simulink model "Test_control_Openfast"  (R2021b)
settings: Solver=ode4  StartTime=0.0  StopTime=TMax  FixedStep=DT  MaxStep=DT  RelTol=1e-3  EnableMultiTasking=on
values from neighbouring files (symbols this model uses):
  Bdt = 4.83e8    (= 483000000)    [Run_Test_control_Openfast.m]
  GBRatio = 87,965    [Run_Test_control_Openfast.m]
  Lambda_opt = 6.443736553192139    (= 6.44373655319)    [Run_Test_control_Openfast.m]
undefined symbols (not defined in the file or in its folder): OutList, strmatch
settings Model: Creator=bjonkman  LastModifiedBy=manip
settings SolverCC: AlgebraicLoopSolver=TrustRegion
settings DataIOCC: LimitDataPoints=on  SignalLoggingSaveFormat=ModelDataLogs  SaveOutput=off  SaveTime=off  ReturnWorkspaceOutputs=off  SignalLoggingName=sigsOut
settings OptimizationCC: ExpressionDepthLimit=2147483647  LifeSpan=inf
settings DebuggingCC: SaveWithParameterizedLinksMsg=none  UnderspecifiedInitializationDetection=Classic  MergeDetectMultiDrivingBlocksExec=none  SignalResolutionControl=TryResolveAllWithWarning  MultiTaskDSMMsg=warning  MultiTaskCondExecSysMsg=none  MultiTaskRateTransMsg=warning  FcnCallInpInsideContextMsg=warning  StateNameClashWarn=warning  SFUnexpectedBacktrackingDiag=warning  SFNoUnconditionalDefaultTransitionDiag=warning  SFExecutionAtInitializationDiag=none  SFMachineParentedDataDiag=warning  ArithmeticOperatorsInVariantConditions=warning
settings HardwareCC: ProdBitPerPointer=32  ProdBitPerSizeT=32  ProdBitPerPtrDiffT=32  ProdLargestAtomicFloat=None  ProdIntDivRoundTo=Undefined  ProdEndianess=Unspecified  ProdWordSize=32  ProdHWDeviceType=32-bit Generic  TargetUnknown=on
settings ModelReferenceCC: PropagateSignalLabelsOutOfModel=off
settings SFSimCC: SimUseLocalCustomCode=off  CustomCodeUndefinedFunction=UseInterfaceOnly
settings RTWCC: RTWUseLocalCustomCode=off
settings CodeAppCC: StateflowObjectComments=on
settings GRTTargetCC: TargetLangStandard=C89/C90 (ANSI)  CombineOutputUpdateFcns=off  GRTInterface=on
settings ConfigComp: CovMetricSettings=dw  CovSaveCumulativeToWorkspaceVar=on  CovSaveSingleToWorkspaceVar=on  CovExternalEMLEnable=off

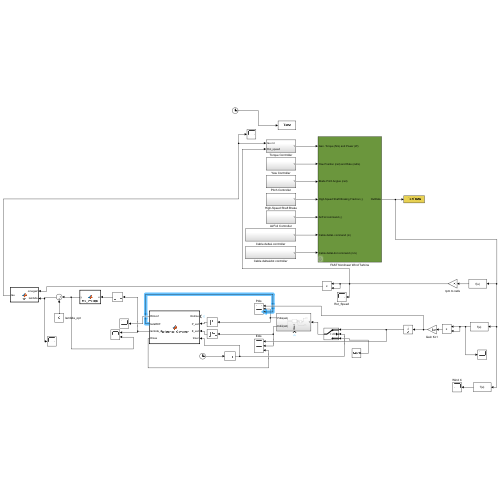
[thumbnail: Simulink's stored preview of the top-level diagram]
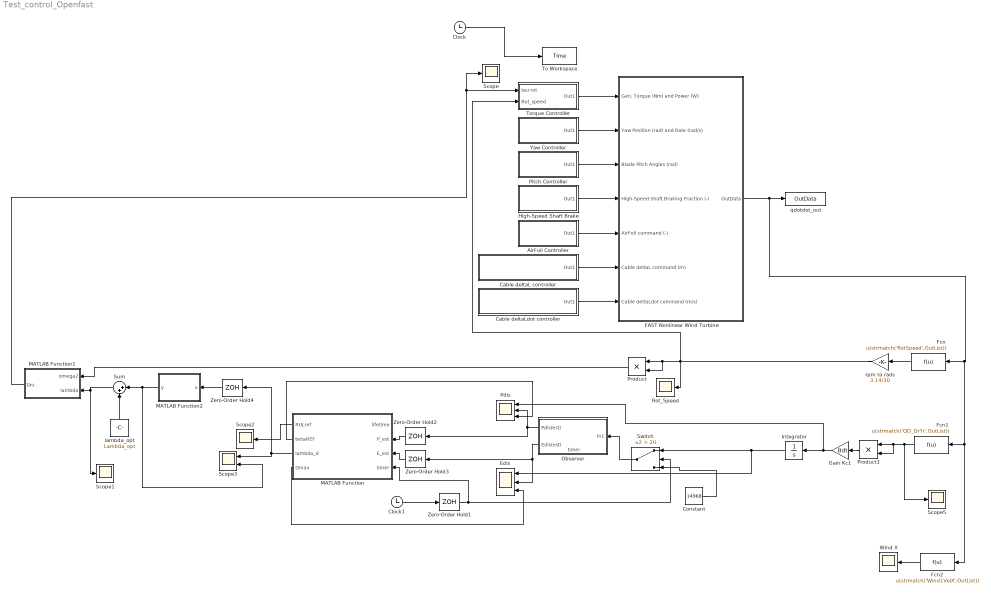
== system Test_control_Openfast ==
  AirFoil Controller : Subsystem
  Cable deltaL controller : Subsystem
  Cable deltaLdot controller : Subsystem
  Clock : Clock
  Clock1 : Clock
  Constant : Constant  Value=14968
  Edis : Scope  NumInputPorts=3
  FAST Nonlinear Wind Turbine : Subsystem  mask(FAST Nonlinear Wind Turbine){}
      mask help: This block contains the FAST S-Function.
      mask init:
      | clear FAST_SFunc
  Fcn : Fcn  Expr=u(strmatch('RotSpeed',OutList))
  Fcn1 : Fcn  Expr=u(strmatch('QD_DrTr',OutList))
  Fcn2 : Fcn  Expr=u(strmatch('Wind1VelX',OutList))
  Gain Kc1 : Gain  Gain=Bdt
  High-Speed Shaft Brake : Subsystem
  Integrator : Integrator
  MATLAB Function : MATLAB Function  TreatAsAtomicUnit=on
  MATLAB Function1 : MATLAB Function  TreatAsAtomicUnit=on
  MATLAB Function2 : MATLAB Function  TreatAsAtomicUnit=on
  Observer : Subsystem
      settings: PortSchema="{\"entries\":[{\"content\":{\"sides\":[{\"content\":{\"connectorIds\":[\"In1\"]},\"type\":\"ConnectorPlacement.EquallySpacedRectSide\",\"uuid\":\"45431176-5fec-4c34-81d0-337d69ca9793\"},{\"content\":{\"connectorIds\":[\"Out1\",\"Out2\"],\"side\":\"RIGHT\"},\"type\":\"ConnectorPlacement.EquallySpacedRectSide\",\"uuid\":\"e3405e5b-b033-438f-b194-16e352d87631\"},{\"content\":{\"connectorIds\":[],\"side\":\"TOP\"},\"type\":\"ConnectorPlacement.EquallySpacedRectSide\",\"uuid\":\"639d392e-3d04-4bae-853f-d03d3019a83c\"},{\"content\":{\"connectorIds\":[\"In2\"],\"side\":\"BOTTOM\"},\"type\":\"ConnectorPlacement.EquallySpacedRectSide\",\"uuid\":\"dfd43518-24a4-48aa-b01e-37d00dba9bed\"}]},\"type\":\"ConnectorPlacement.EquallySpacedConnector\",\"uuid\":\"4ac14b68-7214-4060-a02f-334c8370bb31\"}],\"packageUris\":[\"http://schema.mathworks.com/mf0/Connector/R2020b\"],\"version\":\"1.0\"}"
  Pdis : Scope  NumInputPorts=3
  Pitch Controller : Subsystem
  Product : Product
  Product1 : Product
  Rot_Speed : Scope
  Scope{,1..2,5} (4 alike) : Scope
  Scope3 : Scope  NumInputPorts=2
  Sum : Sum  Inputs=|++
  Switch : Switch  Criteria=u2 > Threshold  Threshold=20
  To Workspace : ToWorkspace  VariableName=Time  SampleTime=-1
  Torque Controller : Subsystem
  Wind X : Scope
  Yaw Controller : Subsystem
  Zero-Order Hold1 : ZeroOrderHold
  Zero-Order Hold2 : ZeroOrderHold
  Zero-Order Hold3 : ZeroOrderHold
  Zero-Order Hold4 : ZeroOrderHold  SampleTime=0.005
  "lambda_opt\t" : Constant  Value=Lambda_opt
  qdotdot_out : ToWorkspace  VariableName=OutData  SampleTime=-1
  rpm to rads : Gain  Gain=3.14/30
  wires:
  Clock/1 -> To Workspace/1
  Torque Controller/1(Out1) -> FAST Nonlinear Wind Turbine/1(Gen. Torque (Nm) and Power (W))
  Yaw Controller/1(Out1) -> FAST Nonlinear Wind Turbine/2(Yaw Position (rad) and Rate (rad/s))
  Pitch Controller/1(Out1) -> FAST Nonlinear Wind Turbine/3(Blade Pitch Angles (rad))
  High-Speed Shaft Brake/1(Out1) -> FAST Nonlinear Wind Turbine/4(High-Speed Shaft Braking Fraction (-))
  AirFoil Controller/1(Out1) -> FAST Nonlinear Wind Turbine/5(AirFoil command (-))
  Cable deltaL controller/1(Out1) -> FAST Nonlinear Wind Turbine/6(Cable deltaL command (m))
  Cable deltaLdot controller/1(Out1) -> FAST Nonlinear Wind Turbine/7(Cable deltaLdot command (m/s))
  MATLAB Function1/1(tau) -> Torque Controller/1(tau rot), Scope/1
  Product/1 -> MATLAB Function1/1(omega2)
  FAST Nonlinear Wind Turbine/1(OutData) -> Fcn2/1, Fcn1/1, Fcn/1, qdotdot_out/1
  Fcn/1 -> rpm to rads/1
  rpm to rads/1 -> Product/1, Product/2, Rot_Speed/1, Torque Controller/2(Rot_speed)
  Fcn1/1 -> Scope5/1, Product1/2, Product1/1
  Product1/1 -> Gain Kc1/1
  Observer/1(Pdis(est)) -> Zero-Order Hold2/1, Pdis/2
  "lambda_opt\t"/1 -> Sum/2
  Clock1/1 -> Zero-Order Hold1/1
  Zero-Order Hold1/1 -> Switch/2, MATLAB Function/4(timer)
  MATLAB Function/1(RULref) -> Scope2/1
  MATLAB Function/3(lambda_d) -> Zero-Order Hold4/1, Scope3/1
  Switch/1 -> Observer/1(In1)
  Constant/1 -> Switch/3
  Zero-Order Hold2/1 -> MATLAB Function/2(P_est)
  Zero-Order Hold3/1 -> MATLAB Function/3(E_est)
  Observer/2(Edis(est)) -> Edis/2, Zero-Order Hold3/1
  MATLAB Function/2(betaREF) -> Pdis/3
  MATLAB Function/4(Dmax) -> Edis/3
  Gain Kc1/1 -> Pdis/1, Integrator/1
  MATLAB Function2/1(y) -> Sum/1, Scope3/2
  Sum/1 -> Scope1/1, MATLAB Function1/2(lambda)
  Zero-Order Hold4/1 -> MATLAB Function2/1(u)
  Integrator/1 -> Switch/1, Edis/1
  Fcn2/1 -> Wind X/1

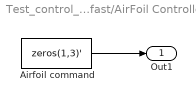
== system Test_control_Openfast/AirFoil Controller ==
  Airfoil command : Constant  Value=zeros(1,3)'
  Out1 : Outport
  wires:
  Airfoil command/1 -> Out1/1

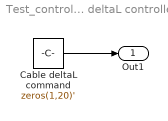
== system Test_control_Openfast/Cable deltaL controller ==
  Cable deltaL command : Constant  Value=zeros(1,20)'
  Out1 : Outport
  wires:
  Cable deltaL command/1 -> Out1/1

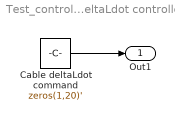
== system Test_control_Openfast/Cable deltaLdot controller ==
  Cable deltaLdot command : Constant  Value=zeros(1,20)'
  Out1 : Outport
  wires:
  Cable deltaLdot command/1 -> Out1/1

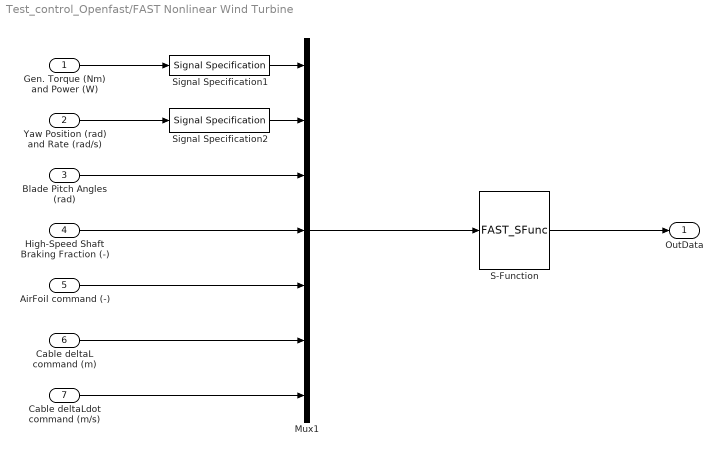
== system Test_control_Openfast/FAST Nonlinear Wind Turbine ==
  Gen. Torque (Nm) and Power (W) : Inport
  Yaw Position (rad) and Rate (rad/s) : Inport  Port=2
  Blade Pitch Angles (rad) : Inport  Port=3
  High-Speed Shaft Braking Fraction (-) : Inport  Port=4
  AirFoil command (-) : Inport  Port=5
  Cable deltaL command (m) : Inport  Port=6
  Cable deltaLdot command (m/s) : Inport  Port=7
  Mux1 : Mux  Inputs=7
  S-Function : S-Function  FunctionName=FAST_SFunc  Parameters=FAST_InputFileName, TMax, 0  SFunctionDeploymentMode=off  EnableBusSupport=off
  Signal Specification1 : SignalSpecification  OutDataTypeStr=double  Dimensions=2
  Signal Specification2 : SignalSpecification  OutDataTypeStr=double  Dimensions=2
  OutData : Outport
  wires:
  Gen. Torque (Nm) and Power (W)/1 -> Signal Specification1/1
  Mux1/1 -> S-Function/1
  Blade Pitch Angles (rad)/1 -> Mux1/3
  Yaw Position (rad) and Rate (rad/s)/1 -> Signal Specification2/1
  Signal Specification1/1 -> Mux1/1
  Signal Specification2/1 -> Mux1/2
  High-Speed Shaft Braking Fraction (-)/1 -> Mux1/4
  AirFoil command (-)/1 -> Mux1/5
  Cable deltaL command (m)/1 -> Mux1/6
  Cable deltaLdot command (m/s)/1 -> Mux1/7
  S-Function/1 -> OutData/1

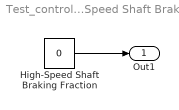
== system Test_control_Openfast/High-Speed Shaft Brake ==
  High-Speed Shaft Braking Fraction : Constant  Value=0
  Out1 : Outport
  wires:
  High-Speed Shaft Braking Fraction/1 -> Out1/1

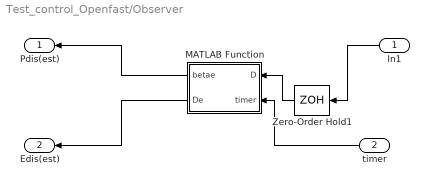
== system Test_control_Openfast/Observer ==
  In1 : Inport
  timer : Inport  Port=2
  MATLAB Function : MATLAB Function  TreatAsAtomicUnit=on
  Zero-Order Hold1 : ZeroOrderHold
  Pdis(est) : Outport
  Edis(est) : Outport  Port=2
  wires:
  Zero-Order Hold1/1 -> MATLAB Function/1(D)
  MATLAB Function/1(betae) -> Pdis(est)/1
  MATLAB Function/2(De) -> Edis(est)/1
  In1/1 -> Zero-Order Hold1/1
  timer/1 -> MATLAB Function/2(timer)

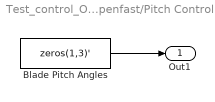
== system Test_control_Openfast/Pitch Controller ==
  Blade Pitch Angles : Constant  Value=zeros(1,3)'
  Out1 : Outport
  wires:
  Blade Pitch Angles/1 -> Out1/1

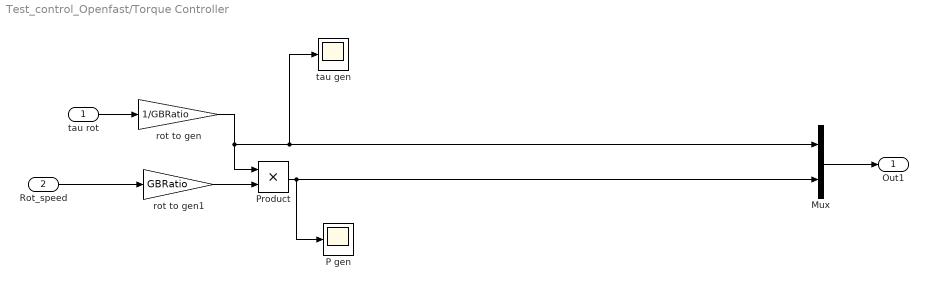
== system Test_control_Openfast/Torque Controller ==
  tau rot : Inport
  Rot_speed : Inport  Port=2
  Mux : Mux  Inputs=2
  P gen : Scope
  Product : Product
  rot to gen : Gain  Gain=1/GBRatio
  rot to gen1 : Gain  Gain=GBRatio
  tau gen : Scope
  Out1 : Outport
  wires:
  Rot_speed/1 -> rot to gen1/1
  Mux/1 -> Out1/1
  rot to gen/1 -> Mux/1, tau gen/1, Product/1
  Product/1 -> Mux/2, P gen/1
  tau rot/1 -> rot to gen/1
  rot to gen1/1 -> Product/2

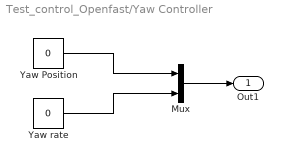
== system Test_control_Openfast/Yaw Controller ==
  Mux : Mux  Inputs=2
  Yaw Position : Constant  Value=0
  Yaw rate : Constant  Value=0
  Out1 : Outport
  wires:
  Mux/1 -> Out1/1
  Yaw Position/1 -> Mux/1
  Yaw rate/1 -> Mux/2

== matlab function Test_control_Openfast/MATLAB Function1 ==
  data: omega2 input; lambda input; tau output
function tau = fcn(omega2,lambda)
rho_air=1.225;
R_r=70/2;
A=pi*R_r*R_r;
Cpmax=0.465813666582108;
k=0.5*rho_air*A*R_r*R_r*R_r*Cpmax/(lambda*lambda*lambda);
tau = k*omega2;

== matlab function Test_control_Openfast/Observer/MATLAB Function ==
  data: D input; betae output; De output; timer input
function [betae,De] = Observer(D,timer)
persistent x P

%%%%%%%%%%%%%%%%%%%%%%%%%%%%
if isempty(x)   
    % initial deterioration: 
    x=[14968;1];
end
if isempty(P)    
    P=[100 0;
       0 10];
end

Ts=1; c=0; 
Q=[10 0; 0 2.5]; %0*(0.05/100)^2];
R=10;
%%%%%%%%%%%%%%%%%%%%%%%%%%%%

    De = x(1); %estimated deterioration
    betae = x(2); %estimated beta

    noise = 0;%0.1*randn(1);
    y = abs(D + noise); %sensor (D has to be an strictly positive mesure)
    
    Ac = [0  1;
          0 -c];
       
    A = eye(2)+Ts*Ac ;  %Euler approximation 
    %A = expm(Ac*Ts);  %Exact solution (for comparison)
    
    C=[1 0];
    
    P = A*P*A'+Q;
    K = P*C'*inv(C*P*C'+R);
    P=(eye(2)-K*C)*P;

    error=(y - C*x);
    
    x1 = A*x + K*error;

    if x(1)< 0, x(1)=0; end
    if x(2)< 0, x(2)=0; end
    
    De = x(1); %estimated deterioration
    betae = x(2); %estimated beta

    %update:
    x=x1;

== matlab function Test_control_Openfast/MATLAB Function ==
  data: lifetime input; RULref output; P_est input; E_est input; timer input; betaREF output; lambda_d output; Dmax output
function [RULref,betaREF,lambda_d,Dmax]  = Reference_Governor(lifetime,P_est,E_est,timer)

persistent z lambda_d_old

if isempty(z)   
    % initial deterioration: 
    lambda_d_old = 0;
    
    K1=0.4460;
    K2=0.07443;

    z=(lambda_d_old+K1*lambda_d_old)/-K2;

    
end
K1=0.4460;
K2=0.07443;


Ts=1;

%RUL reference generation:
Lifetime = 500;
RULref=-1*timer+Lifetime;

%References for parameter beta
Dmax=1.499e4; %Admissible max deterioration

%RUL_min= (Dmax-Dt)/0.2859;
%RUL_max= (Dmax-Dt)/9.7e-5;

%if RULref < RUL_min
 %   RULref= RUL_min;
%end

%if RULref > RUL_max
 %   RULref= RUL_max;
%end

if RULref < 1
    RULref= 1;
end


if timer > 30
betaREF = (Dmax-E_est)/RULref;

z = z + Ts*(P_est-betaREF);

%Find optimal decision:
wref = -K1*lambda_d_old - K2*z ;

%The optimal decision at time k
lambda_d =lambda_d_old;

%update the decision for next step iteration:
lambda_d_old = wref;
else

betaREF =0/RULref;

z = z + Ts*(0);

%Find optimal decision:
wref = 0 ;

%The optimal decision at time k
lambda_d =lambda_d_old;

%update the decision for next step iteration:
lambda_d_old = wref;
end
%%%%%%%%%%%%%%%%%%

== matlab function Test_control_Openfast/MATLAB Function2 ==
  data: u input; y output
function y = my_average(u) %# codegen
persistent i buf bufSum;
if isempty(buf)
    buf = zeros(1,200);
    bufSum = 0;
    i = 1;
end
bufSum = bufSum - buf(i);
buf(i) = u;
bufSum = bufSum + u;
i = i + 1;
if i > numel(buf)
    i = 1;
end
y = bufSum / numel(buf);
